simulink model "signal_model"  (R2023a)
settings: Solver=VariableStepAuto  StartTime=0.0  StopTime=10.0  RelTol=1e-3
undefined symbols (not defined in the file or in its folder): phased, physconst
libraries: simrfV2util1 x4, phaseddoalib x2, dspsrcs4 x2, simrfV2systems x1, phasedtxrxlib x1
settings Model: Creator=david  LastModifiedBy=david

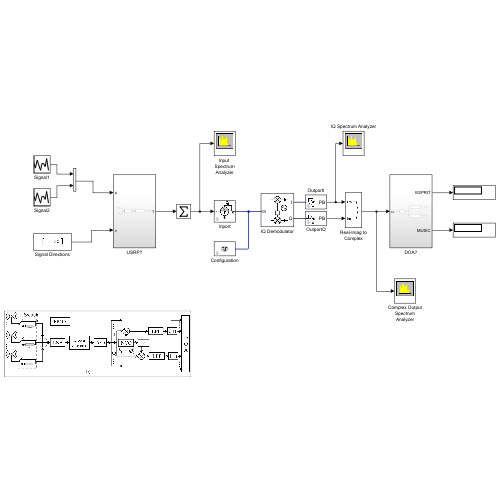
[thumbnail: Simulink's stored preview of the top-level diagram]
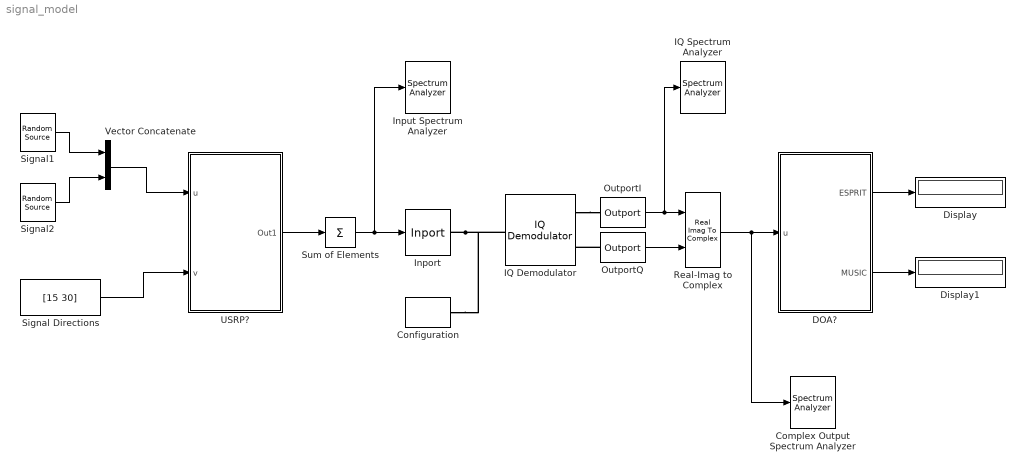
== system signal_model ==
  Complex Output Spectrum Analyzer : SpectrumAnalyzer  WindowPosition=[2871 540 871 495]  ScopeFrameLocation=window  Method=Welch  SampleRate=100000000  AxesScaling=Manual  Span=15360000  StartFrequency=-7680000  StopFrequency=7680000  RBWSource=Property  RBW=1e4  FFTLengthSource=Property  FFTLength=512  WindowLength=512  AveragingMethod=Running  SpectralAverages=10  YLimits=[-158.27120633437067,18.319537380765393]  ShowLegend=on  DefaultConfigurationName=spbscopes.SpectrumAnalyzerBlockCfg  IsFrequencyInputMode=0  FrequencyVectorPort=0  FrequencyVectorFromPort=0  FrequencyInputRBWPort=0  FrequencyInputRBWFromPort=0
      settings: OpenAtSimulationStart=off
  Configuration : simrfV2util1/Configuration  AutoFreq=on  Tones=[2] GHz  Harmonics=[7]  NormalizeCarrierPower=on  SolverType=Auto  UseCCode=on  StepSize=1e-8 s  AddNoise=on  defaultRNG=on  Seed=0  Temperature=290.0 K  SolverDelFlag=0  AbsTol=1e-6  RelTol=1e-3  MaxIter=10  ErrorEstimationType=2-norm over all variables  EnableInterpFilter=off  HiddenFIRfilterControllerParam=on  SmallSignalApprox=off  AllSimFreqs=on  SimFreqs=[] Hz  SimFreqsInternal=[]  SamplesPerFrame=1
  DOA? : Subsystem
  Display : Display
  Display1 : Display
  IQ Demodulator : simrfV2systems/IQ Demodulator  classname=iqdemod  Source_linear_gain=Available power gain  linear_gain=10 dB  Poly_Coeffs=[0 1]  LOFreq=2 GHz  Zin=50  Zout=50  AddIRFilter=off  AddCSFilters=off  InternalGrounding=on  ForceNextInit=off  Source_Poly=Even and odd order  IPType=Output  IP2=inf dBm  IP3=20 dBm  P1dB=inf dBm  Psat=inf dBm  Gcomp=inf dBm  NF=6  GainMismatch=0.1 dB  PhaseMismatch=0 deg  Isolation=90 dB  AddPhaseNoise=off  PhaseNoiseOffset=1  PhaseNoiseLevel=-Inf  AutoImpulseLengthPN=on  ImpulseLengthPN=1e-10  ImpulseLength_unitPN=s  DesignMethodIR=Ideal  ResponseTypeIR=Highpass  ImplementationIR=LC Tee  ImplementationIdealIR=Constant per carrier  ImplementationRationalIR=Transfer function  UseFilterOrderIR=on  FilterOrderIR=3  PassFreq_lpIR=1  PassFreq_lp_unitIR=GHz  PassFreq_hpIR=2  PassFreq_hp_unitIR=GHz  PassFreq_bpIR=[2 3]  PassFreq_bp_unitIR=GHz  PassFreq_bsIR=[1 4]  PassFreq_bs_unitIR=GHz  PassAttenIR=10*log10(2)  StopFreq_lpIR=2  StopFreq_lp_unitIR=GHz  StopFreq_hpIR=1  StopFreq_hp_unitIR=GHz  StopFreq_bpIR=[1.5 3.5]  StopFreq_bp_unitIR=GHz  StopFreq_bsIR=[2.1 2.9]  StopFreq_bs_unitIR=GHz  StopAttenIR=40  RsrcIR=50  RloadIR=50  AutoImpulseLengthIR=on  ImpulseLengthIR=1e-10  ImpulseLength_unitIR=s  DesignMethodCS=Ideal  ResponseTypeCS=Lowpass  ImplementationCS=LC Tee  ImplementationIdealCS=Constant per carrier  ImplementationRationalCS=Transfer function  UseFilterOrderCS=on  FilterOrderCS=3  PassFreq_lpCS=1  PassFreq_lp_unitCS=GHz  PassFreq_hpCS=2  PassFreq_hp_unitCS=GHz  PassFreq_bpCS=[2 3]  PassFreq_bp_unitCS=GHz  PassFreq_bsCS=[1 4]  PassFreq_bs_unitCS=GHz  PassAttenCS=10*log10(2)  StopFreq_lpCS=2  StopFreq_lp_unitCS=GHz  StopFreq_hpCS=1  StopFreq_hp_unitCS=GHz  StopFreq_bpCS=[1.5 3.5]  StopFreq_bp_unitCS=GHz  StopFreq_bsCS=[2.1 2.9]  StopFreq_bs_unitCS=GHz  StopAttenCS=40  RsrcCS=50  RloadCS=50  AutoImpulseLengthCS=on  ImpulseLengthCS=1e-10  ImpulseLength_unitCS=s
  IQ Spectrum Analyzer : SpectrumAnalyzer  WindowPosition=[695 477 863 492]  ScopeFrameLocation=window  Method=Welch  SampleRate=100000000  PlotAsTwoSidedSpectrum=off  AxesScaling=Manual  Span=15360000  StartFrequency=-7680000  StopFrequency=7680000  RBWSource=Property  RBW=1e4  FFTLengthSource=Property  FFTLength=512  WindowLength=512  AveragingMethod=Running  SpectralAverages=10  YLimits=[-207.59950539890519,30.660365661921674]  ShowLegend=on  DefaultConfigurationName=spbscopes.SpectrumAnalyzerBlockCfg  IsFrequencyInputMode=0  FrequencyVectorPort=0  FrequencyVectorFromPort=0  FrequencyInputRBWPort=0  FrequencyInputRBWFromPort=0
      settings: OpenAtSimulationStart=off
  Inport : simrfV2util1/Inport  SimulinkInputSignalType=Power  CarrierFreq=2 GHz  ZS=50  UseSqWave=off  NumCoeff=10  Bias=0  DutyCyc=50  InternalGrounding=on
  "Input Spectrum Analyzer " : SpectrumAnalyzer  WindowPosition=[114 465 868 508]  ScopeFrameLocation=window  Method=Welch  SampleRate=100000000  AxesScaling=Manual  Span=15360000  StartFrequency=-7680000  StopFrequency=7680000  RBW=1e4  FFTLengthSource=Property  FFTLength=512  WindowLength=512  AveragingMethod=Running  SpectralAverages=10  YLimits=[-304.77978506317356,-6.2207505227562834]  ShowLegend=on  DefaultConfigurationName=spbscopes.SpectrumAnalyzerBlockCfg  IsFrequencyInputMode=0  FrequencyVectorPort=0  FrequencyVectorFromPort=0  FrequencyInputRBWPort=0  FrequencyInputRBWFromPort=0
      settings: OpenAtSimulationStart=off
  OutportI : simrfV2util1/Outport  SensorType=Power  OutputFormat=Real Passband  CarrierFreq=0 GHz  ZL=50  InternalGrounding=on  StepSize=-1 s  AutoStep=off  HalfPolyphaseLength=0
  OutportQ : simrfV2util1/Outport  SensorType=Power  OutputFormat=Real Passband  CarrierFreq=0 GHz  ZL=50  InternalGrounding=on  StepSize=-1 s  AutoStep=off  HalfPolyphaseLength=0
  Real-Imag to Complex : RealImagToComplex
  Signal Directions : Constant  Value=[15 30]
  Signal1 : dspsrcs4/Random Source  SrcType=Gaussian  NormMethod=Ziggurat  CltLength=12  MinVal=0  MaxVal=1  MeanVal=0  VarVal=100  RepMode=Repeatable  rawSeed=1  IsInherit=off  SampMode=Discrete  SampTime=1/1000  SampFrame=1000  DataType=Double  OutComplex=Real  OutputFrames=on
  Signal2 : dspsrcs4/Random Source  SrcType=Gaussian  NormMethod=Ziggurat  CltLength=12  MinVal=0  MaxVal=1  MeanVal=0  VarVal=50  RepMode=Repeatable  rawSeed=1  IsInherit=off  SampMode=Discrete  SampTime=1/1000  SampFrame=1000  DataType=Double  OutComplex=Real  OutputFrames=on
  Sum of Elements : Sum  Inputs=+
  USRP? : Subsystem
  Vector Concatenate : Concatenate  Mode=Multidimensional array  ConcatenateDimension=2
  wires:
  OutportQ/1 -> Real-Imag to Complex/2
  Sum of Elements/1 -> "Input Spectrum Analyzer "/1, Inport/1
  OutportI/1 -> Real-Imag to Complex/1, IQ Spectrum Analyzer/1
  Real-Imag to Complex/1 -> Complex Output Spectrum Analyzer/1, DOA?/1(u)
  USRP?/1(Out1) -> Sum of Elements/1
  Signal1/1 -> Vector Concatenate/1
  Signal2/1 -> Vector Concatenate/2
  Vector Concatenate/1 -> USRP?/1(u)
  Signal Directions/1 -> USRP?/2(v)
  DOA?/1(ESPRIT) -> Display/1
  DOA?/2(MUSIC) -> Display1/1
  connections:
  Inport/RConn1 -- Configuration/LConn1 -- IQ Demodulator/LConn1
  OutportQ/LConn1 -- IQ Demodulator/RConn2
  IQ Demodulator/RConn1 -- OutportI/LConn1

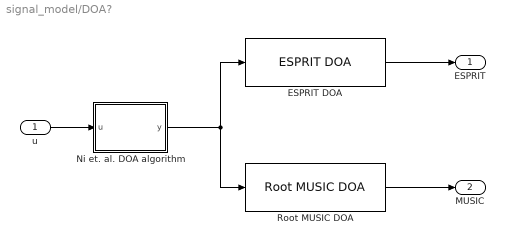
== system signal_model/DOA? ==
  u : Inport
  ESPRIT DOA : phaseddoalib/ESPRIT DOA  PropagationSpeed=physconst( 'LightSpeed' )  OperatingFrequency=3e8  NumSignalsSource=Property  NumSignalsMethod=AIC  NumSignals=1  SpatialSmoothing=0  Method=TLS  ForwardBackwardAveraging=off  RowWeighting=1  SimulateUsing=Interpreted execution  SensorArray=phased.ULA('Element',phased.IsotropicAntennaElement)
  Ni et. al. DOA algorithm : MATLAB Function  TreatAsAtomicUnit=on
  Root MUSIC DOA : phaseddoalib/Root MUSIC DOA  PropagationSpeed=physconst( 'LightSpeed' )  OperatingFrequency=3e8  NumSignalsSource=Property  NumSignalsMethod=AIC  NumSignals=1  ForwardBackwardAveraging=off  SpatialSmoothing=0  SimulateUsing=Interpreted execution  SensorArray=phased.ULA('Element',phased.IsotropicAntennaElement)
  ESPRIT : Outport
  MUSIC : Outport  Port=2
  wires:
  u/1 -> Ni et. al. DOA algorithm/1(u)
  Ni et. al. DOA algorithm/1(y) -> Root MUSIC DOA/1, ESPRIT DOA/1
  ESPRIT DOA/1 -> ESPRIT/1
  Root MUSIC DOA/1 -> MUSIC/1

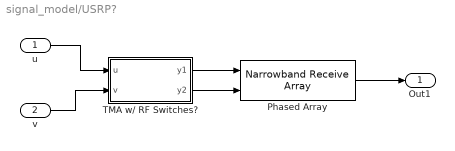
== system signal_model/USRP? ==
  u : Inport
  v : Inport  Port=2
  "Phased Array " : phasedtxrxlib/Narrowband Receive Array  PropagationSpeed=physconst( 'LightSpeed' )  OperatingFrequency=3e8  Wavefront=Plane  SensorGainMeasure=dB  Polarization=None  WeightsInputPort=off  SimulateUsing=Interpreted execution  Sensor=phased.ULA('Element',phased.IsotropicAntennaElement)
  TMA w/ RF Switches? : MATLAB Function  TreatAsAtomicUnit=on
  Out1 : Outport
  wires:
  "Phased Array "/1 -> Out1/1
  v/1 -> TMA w/ RF Switches?/2(v)
  u/1 -> TMA w/ RF Switches?/1(u)
  TMA w/ RF Switches?/1(y1) -> "Phased Array "/1
  TMA w/ RF Switches?/2(y2) -> "Phased Array "/2

== matlab function signal_model/DOA?/Ni et. al. DOA algorithm ==
  data: u input; y output
function y = fcn(u)

y = u;

== matlab function signal_model/USRP?/TMA w// RF Switches? ==
  data: u input; y1 output; v input; y2 output
function [y1, y2]= fcn(u, v)

y2 = u;
